simulink model "VGrowth4"  (R2018b)
settings: Solver=VariableStepAuto  StartTime=0.0  StopTime=12  RelTol=1e-3
libraries: simulink x1
settings Model: Creator=Magneto  LastModifiedBy=Magneto

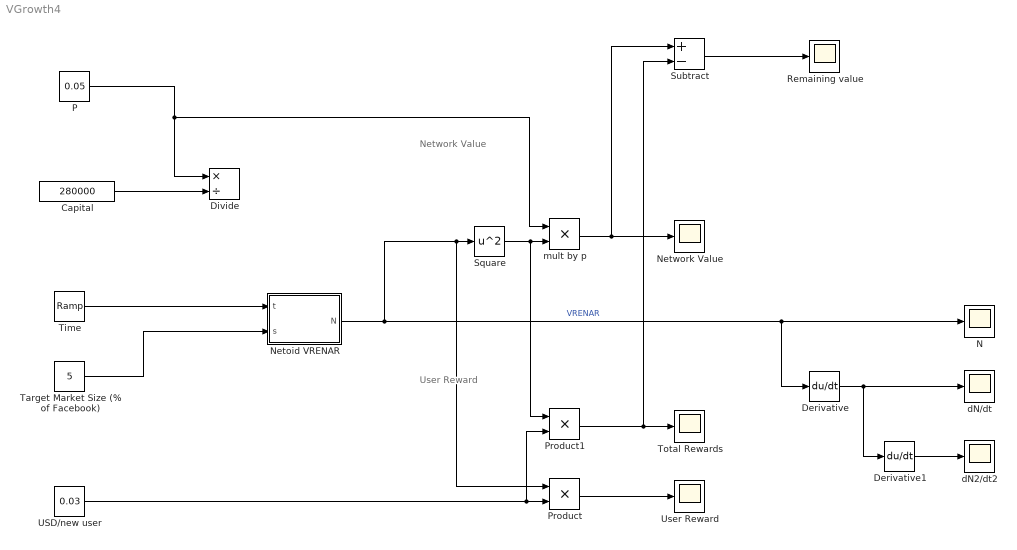
== system VGrowth4 ==
  note: User Reward
  note: Network Value
  Capital : Constant  Value=280000
  Derivative : Derivative
  Derivative1 : Derivative
  Divide : Product  Inputs=*/
  N : Scope
  Netoid VRENAR : MATLAB Function  TreatAsAtomicUnit=on
  Network Value : Scope
  P : Constant  Value=0.05
  Product : Product
  Product1 : Product
  Remaining value : Scope
  Square : Math  Operator=square  SaturateOnIntegerOverflow=on
  Subtract : Sum  Inputs=+-
  Target Market Size (% of Facebook) : Constant  Value=5
  Time : simulink/Sources/Ramp  slope=1  start=0  InitialOutput=0
  Total Rewards : Scope
  USD/new user : Constant  Value=0.03
  User Reward : Scope
  dN/dt : Scope
  dN2/dt2 : Scope
  mult by p : Product
  wires:
  Time/1 -> Netoid VRENAR/1(t)
  Target Market Size (% of Facebook)/1 -> Netoid VRENAR/2(s)
  Netoid VRENAR/1(N) -> Product/1, Square/1, Derivative/1, N/1  "VRENAR"
  Square/1 -> Product1/1, mult by p/2
  mult by p/1 -> Subtract/1, Network Value/1
  Capital/1 -> Divide/2
  USD/new user/1 -> Product1/2, Product/2
  Product/1 -> User Reward/1
  P/1 -> mult by p/1, Divide/1
  Product1/1 -> Total Rewards/1, Subtract/2
  Subtract/1 -> Remaining value/1
  Derivative/1 -> Derivative1/1, dN/dt/1
  Derivative1/1 -> dN2/dt2/1

== matlab function VGrowth4/Netoid VRENAR ==
  data: t input; N output; s input
function N = fcn(t,s)

% Additional term -(1.45e9/(1+exp(-1.155*(-5)))) added to initialise N
% closer to zero at t=0
N = (s/100)*(1.45e9*((1/(1+exp(-1.155*(t-5))))-(1/(1+exp(-1.155*(-5))))));
